simulink model "receiver_overall_reset"  (Simulink 7.5)
settings: Solver=FixedStepDiscrete  SolverMode=SingleTasking  StartTime=0.0  StopTime=(length(simin.signals.values)-1)/Fs  FixedStep=1  RelTol=1e-3
undefined symbols (not defined in the file): Fs
libraries: xbsIndex_r4 x962
(part 9 of 9)

== system receiver_overall_reset/Receiver/Sym-Chooser/3-11/Corr0/Delay_Line/DE14/1to2 ==
  In : Inport  OutDataType=fixdt(1, 16)  OutScaling=2^0
  Out1 : Outport  OutDataType=fixdt(1, 16)  OutScaling=2^0
  Out2 : Outport  Port=2  OutDataType=fixdt(1, 16)  OutScaling=2^0
  wires:
  In/1 -> Out2/1, Out1/1

== system receiver_overall_reset/Receiver/Sym-Chooser/3-11/Corr0/Delay_Line/DE15/1to2 ==
  In : Inport  OutDataType=fixdt(1, 16)  OutScaling=2^0
  Out1 : Outport  OutDataType=fixdt(1, 16)  OutScaling=2^0
  Out2 : Outport  Port=2  OutDataType=fixdt(1, 16)  OutScaling=2^0
  wires:
  In/1 -> Out2/1, Out1/1

== system receiver_overall_reset/Receiver/Sym-Chooser/3-11/Corr0/Delay_Line/DE16/1to2 ==
  In : Inport  OutDataType=fixdt(1, 16)  OutScaling=2^0
  Out1 : Outport  OutDataType=fixdt(1, 16)  OutScaling=2^0
  Out2 : Outport  Port=2  OutDataType=fixdt(1, 16)  OutScaling=2^0
  wires:
  In/1 -> Out2/1, Out1/1

== system receiver_overall_reset/Receiver/Sym-Chooser/3-11/Corr0/Delay_Line/DE17/1to2 ==
  In : Inport  OutDataType=fixdt(1, 16)  OutScaling=2^0
  Out1 : Outport  OutDataType=fixdt(1, 16)  OutScaling=2^0
  Out2 : Outport  Port=2  OutDataType=fixdt(1, 16)  OutScaling=2^0
  wires:
  In/1 -> Out2/1, Out1/1

== system receiver_overall_reset/Receiver/Sym-Chooser/3-11/Corr0/Delay_Line/DE18/1to2 ==
  In : Inport  OutDataType=fixdt(1, 16)  OutScaling=2^0
  Out1 : Outport  OutDataType=fixdt(1, 16)  OutScaling=2^0
  Out2 : Outport  Port=2  OutDataType=fixdt(1, 16)  OutScaling=2^0
  wires:
  In/1 -> Out2/1, Out1/1

== system receiver_overall_reset/Receiver/Sym-Chooser/3-11/Corr0/Delay_Line/DE19/1to2 ==
  In : Inport  OutDataType=fixdt(1, 16)  OutScaling=2^0
  Out1 : Outport  OutDataType=fixdt(1, 16)  OutScaling=2^0
  Out2 : Outport  Port=2  OutDataType=fixdt(1, 16)  OutScaling=2^0
  wires:
  In/1 -> Out2/1, Out1/1

== system receiver_overall_reset/Receiver/Sym-Chooser/3-11/Corr0/Delay_Line/DE2/1to2 ==
  In : Inport  OutDataType=fixdt(1, 16)  OutScaling=2^0
  Out1 : Outport  OutDataType=fixdt(1, 16)  OutScaling=2^0
  Out2 : Outport  Port=2  OutDataType=fixdt(1, 16)  OutScaling=2^0
  wires:
  In/1 -> Out2/1, Out1/1

== system receiver_overall_reset/Receiver/Sym-Chooser/3-11/Corr0/Delay_Line/DE20/1to2 ==
  In : Inport  OutDataType=fixdt(1, 16)  OutScaling=2^0
  Out1 : Outport  OutDataType=fixdt(1, 16)  OutScaling=2^0
  Out2 : Outport  Port=2  OutDataType=fixdt(1, 16)  OutScaling=2^0
  wires:
  In/1 -> Out2/1, Out1/1

== system receiver_overall_reset/Receiver/Sym-Chooser/3-11/Corr0/Delay_Line/DE21/1to2 ==
  In : Inport  OutDataType=fixdt(1, 16)  OutScaling=2^0
  Out1 : Outport  OutDataType=fixdt(1, 16)  OutScaling=2^0
  Out2 : Outport  Port=2  OutDataType=fixdt(1, 16)  OutScaling=2^0
  wires:
  In/1 -> Out2/1, Out1/1

== system receiver_overall_reset/Receiver/Sym-Chooser/3-11/Corr0/Delay_Line/DE22/1to2 ==
  In : Inport  OutDataType=fixdt(1, 16)  OutScaling=2^0
  Out1 : Outport  OutDataType=fixdt(1, 16)  OutScaling=2^0
  Out2 : Outport  Port=2  OutDataType=fixdt(1, 16)  OutScaling=2^0
  wires:
  In/1 -> Out2/1, Out1/1

== system receiver_overall_reset/Receiver/Sym-Chooser/3-11/Corr0/Delay_Line/DE23/1to2 ==
  In : Inport  OutDataType=fixdt(1, 16)  OutScaling=2^0
  Out1 : Outport  OutDataType=fixdt(1, 16)  OutScaling=2^0
  Out2 : Outport  Port=2  OutDataType=fixdt(1, 16)  OutScaling=2^0
  wires:
  In/1 -> Out2/1, Out1/1

== system receiver_overall_reset/Receiver/Sym-Chooser/3-11/Corr0/Delay_Line/DE24/1to2 ==
  In : Inport  OutDataType=fixdt(1, 16)  OutScaling=2^0
  Out1 : Outport  OutDataType=fixdt(1, 16)  OutScaling=2^0
  Out2 : Outport  Port=2  OutDataType=fixdt(1, 16)  OutScaling=2^0
  wires:
  In/1 -> Out2/1, Out1/1

== system receiver_overall_reset/Receiver/Sym-Chooser/3-11/Corr0/Delay_Line/DE25/1to2 ==
  In : Inport  OutDataType=fixdt(1, 16)  OutScaling=2^0
  Out1 : Outport  OutDataType=fixdt(1, 16)  OutScaling=2^0
  Out2 : Outport  Port=2  OutDataType=fixdt(1, 16)  OutScaling=2^0
  wires:
  In/1 -> Out2/1, Out1/1

== system receiver_overall_reset/Receiver/Sym-Chooser/3-11/Corr0/Delay_Line/DE26/1to2 ==
  In : Inport  OutDataType=fixdt(1, 16)  OutScaling=2^0
  Out1 : Outport  OutDataType=fixdt(1, 16)  OutScaling=2^0
  Out2 : Outport  Port=2  OutDataType=fixdt(1, 16)  OutScaling=2^0
  wires:
  In/1 -> Out2/1, Out1/1

== system receiver_overall_reset/Receiver/Sym-Chooser/3-11/Corr0/Delay_Line/DE27/1to2 ==
  In : Inport  OutDataType=fixdt(1, 16)  OutScaling=2^0
  Out1 : Outport  OutDataType=fixdt(1, 16)  OutScaling=2^0
  Out2 : Outport  Port=2  OutDataType=fixdt(1, 16)  OutScaling=2^0
  wires:
  In/1 -> Out2/1, Out1/1

== system receiver_overall_reset/Receiver/Sym-Chooser/3-11/Corr0/Delay_Line/DE28/1to2 ==
  In : Inport  OutDataType=fixdt(1, 16)  OutScaling=2^0
  Out1 : Outport  OutDataType=fixdt(1, 16)  OutScaling=2^0
  Out2 : Outport  Port=2  OutDataType=fixdt(1, 16)  OutScaling=2^0
  wires:
  In/1 -> Out2/1, Out1/1

== system receiver_overall_reset/Receiver/Sym-Chooser/3-11/Corr0/Delay_Line/DE29/1to2 ==
  In : Inport  OutDataType=fixdt(1, 16)  OutScaling=2^0
  Out1 : Outport  OutDataType=fixdt(1, 16)  OutScaling=2^0
  Out2 : Outport  Port=2  OutDataType=fixdt(1, 16)  OutScaling=2^0
  wires:
  In/1 -> Out2/1, Out1/1

== system receiver_overall_reset/Receiver/Sym-Chooser/3-11/Corr0/Delay_Line/DE3/1to2 ==
  In : Inport  OutDataType=fixdt(1, 16)  OutScaling=2^0
  Out1 : Outport  OutDataType=fixdt(1, 16)  OutScaling=2^0
  Out2 : Outport  Port=2  OutDataType=fixdt(1, 16)  OutScaling=2^0
  wires:
  In/1 -> Out2/1, Out1/1

== system receiver_overall_reset/Receiver/Sym-Chooser/3-11/Corr0/Delay_Line/DE30/1to2 ==
  In : Inport  OutDataType=fixdt(1, 16)  OutScaling=2^0
  Out1 : Outport  OutDataType=fixdt(1, 16)  OutScaling=2^0
  Out2 : Outport  Port=2  OutDataType=fixdt(1, 16)  OutScaling=2^0
  wires:
  In/1 -> Out2/1, Out1/1

== system receiver_overall_reset/Receiver/Sym-Chooser/3-11/Corr0/Delay_Line/DE4/1to2 ==
  In : Inport  OutDataType=fixdt(1, 16)  OutScaling=2^0
  Out1 : Outport  OutDataType=fixdt(1, 16)  OutScaling=2^0
  Out2 : Outport  Port=2  OutDataType=fixdt(1, 16)  OutScaling=2^0
  wires:
  In/1 -> Out2/1, Out1/1

== system receiver_overall_reset/Receiver/Sym-Chooser/3-11/Corr0/Delay_Line/DE5/1to2 ==
  In : Inport  OutDataType=fixdt(1, 16)  OutScaling=2^0
  Out1 : Outport  OutDataType=fixdt(1, 16)  OutScaling=2^0
  Out2 : Outport  Port=2  OutDataType=fixdt(1, 16)  OutScaling=2^0
  wires:
  In/1 -> Out2/1, Out1/1

== system receiver_overall_reset/Receiver/Sym-Chooser/3-11/Corr0/Delay_Line/DE6/1to2 ==
  In : Inport  OutDataType=fixdt(1, 16)  OutScaling=2^0
  Out1 : Outport  OutDataType=fixdt(1, 16)  OutScaling=2^0
  Out2 : Outport  Port=2  OutDataType=fixdt(1, 16)  OutScaling=2^0
  wires:
  In/1 -> Out2/1, Out1/1

== system receiver_overall_reset/Receiver/Sym-Chooser/3-11/Corr0/Delay_Line/DE7/1to2 ==
  In : Inport  OutDataType=fixdt(1, 16)  OutScaling=2^0
  Out1 : Outport  OutDataType=fixdt(1, 16)  OutScaling=2^0
  Out2 : Outport  Port=2  OutDataType=fixdt(1, 16)  OutScaling=2^0
  wires:
  In/1 -> Out2/1, Out1/1

== system receiver_overall_reset/Receiver/Sym-Chooser/3-11/Corr0/Delay_Line/DE8/1to2 ==
  In : Inport  OutDataType=fixdt(1, 16)  OutScaling=2^0
  Out1 : Outport  OutDataType=fixdt(1, 16)  OutScaling=2^0
  Out2 : Outport  Port=2  OutDataType=fixdt(1, 16)  OutScaling=2^0
  wires:
  In/1 -> Out2/1, Out1/1

== system receiver_overall_reset/Receiver/Sym-Chooser/3-11/Corr0/Delay_Line/DE9/1to2 ==
  In : Inport  OutDataType=fixdt(1, 16)  OutScaling=2^0
  Out1 : Outport  OutDataType=fixdt(1, 16)  OutScaling=2^0
  Out2 : Outport  Port=2  OutDataType=fixdt(1, 16)  OutScaling=2^0
  wires:
  In/1 -> Out2/1, Out1/1

== system receiver_overall_reset/Receiver/Sym-Chooser/4-12/Corr0/Delay_Line/DE1/1to2 ==
  In : Inport  OutDataType=fixdt(1, 16)  OutScaling=2^0
  Out1 : Outport  OutDataType=fixdt(1, 16)  OutScaling=2^0
  Out2 : Outport  Port=2  OutDataType=fixdt(1, 16)  OutScaling=2^0
  wires:
  In/1 -> Out1/1, Out2/1

== system receiver_overall_reset/Receiver/Sym-Chooser/4-12/Corr0/Delay_Line/DE10/1to2 ==
  In : Inport  OutDataType=fixdt(1, 16)  OutScaling=2^0
  Out1 : Outport  OutDataType=fixdt(1, 16)  OutScaling=2^0
  Out2 : Outport  Port=2  OutDataType=fixdt(1, 16)  OutScaling=2^0
  wires:
  In/1 -> Out2/1, Out1/1

== system receiver_overall_reset/Receiver/Sym-Chooser/4-12/Corr0/Delay_Line/DE11/1to2 ==
  In : Inport  OutDataType=fixdt(1, 16)  OutScaling=2^0
  Out1 : Outport  OutDataType=fixdt(1, 16)  OutScaling=2^0
  Out2 : Outport  Port=2  OutDataType=fixdt(1, 16)  OutScaling=2^0
  wires:
  In/1 -> Out2/1, Out1/1

== system receiver_overall_reset/Receiver/Sym-Chooser/4-12/Corr0/Delay_Line/DE12/1to2 ==
  In : Inport  OutDataType=fixdt(1, 16)  OutScaling=2^0
  Out1 : Outport  OutDataType=fixdt(1, 16)  OutScaling=2^0
  Out2 : Outport  Port=2  OutDataType=fixdt(1, 16)  OutScaling=2^0
  wires:
  In/1 -> Out2/1, Out1/1

== system receiver_overall_reset/Receiver/Sym-Chooser/4-12/Corr0/Delay_Line/DE13/1to2 ==
  In : Inport  OutDataType=fixdt(1, 16)  OutScaling=2^0
  Out1 : Outport  OutDataType=fixdt(1, 16)  OutScaling=2^0
  Out2 : Outport  Port=2  OutDataType=fixdt(1, 16)  OutScaling=2^0
  wires:
  In/1 -> Out2/1, Out1/1

== system receiver_overall_reset/Receiver/Sym-Chooser/4-12/Corr0/Delay_Line/DE14/1to2 ==
  In : Inport  OutDataType=fixdt(1, 16)  OutScaling=2^0
  Out1 : Outport  OutDataType=fixdt(1, 16)  OutScaling=2^0
  Out2 : Outport  Port=2  OutDataType=fixdt(1, 16)  OutScaling=2^0
  wires:
  In/1 -> Out2/1, Out1/1

== system receiver_overall_reset/Receiver/Sym-Chooser/4-12/Corr0/Delay_Line/DE15/1to2 ==
  In : Inport  OutDataType=fixdt(1, 16)  OutScaling=2^0
  Out1 : Outport  OutDataType=fixdt(1, 16)  OutScaling=2^0
  Out2 : Outport  Port=2  OutDataType=fixdt(1, 16)  OutScaling=2^0
  wires:
  In/1 -> Out2/1, Out1/1

== system receiver_overall_reset/Receiver/Sym-Chooser/4-12/Corr0/Delay_Line/DE16/1to2 ==
  In : Inport  OutDataType=fixdt(1, 16)  OutScaling=2^0
  Out1 : Outport  OutDataType=fixdt(1, 16)  OutScaling=2^0
  Out2 : Outport  Port=2  OutDataType=fixdt(1, 16)  OutScaling=2^0
  wires:
  In/1 -> Out2/1, Out1/1

== system receiver_overall_reset/Receiver/Sym-Chooser/4-12/Corr0/Delay_Line/DE17/1to2 ==
  In : Inport  OutDataType=fixdt(1, 16)  OutScaling=2^0
  Out1 : Outport  OutDataType=fixdt(1, 16)  OutScaling=2^0
  Out2 : Outport  Port=2  OutDataType=fixdt(1, 16)  OutScaling=2^0
  wires:
  In/1 -> Out2/1, Out1/1

== system receiver_overall_reset/Receiver/Sym-Chooser/4-12/Corr0/Delay_Line/DE18/1to2 ==
  In : Inport  OutDataType=fixdt(1, 16)  OutScaling=2^0
  Out1 : Outport  OutDataType=fixdt(1, 16)  OutScaling=2^0
  Out2 : Outport  Port=2  OutDataType=fixdt(1, 16)  OutScaling=2^0
  wires:
  In/1 -> Out2/1, Out1/1

== system receiver_overall_reset/Receiver/Sym-Chooser/4-12/Corr0/Delay_Line/DE19/1to2 ==
  In : Inport  OutDataType=fixdt(1, 16)  OutScaling=2^0
  Out1 : Outport  OutDataType=fixdt(1, 16)  OutScaling=2^0
  Out2 : Outport  Port=2  OutDataType=fixdt(1, 16)  OutScaling=2^0
  wires:
  In/1 -> Out2/1, Out1/1

== system receiver_overall_reset/Receiver/Sym-Chooser/4-12/Corr0/Delay_Line/DE2/1to2 ==
  In : Inport  OutDataType=fixdt(1, 16)  OutScaling=2^0
  Out1 : Outport  OutDataType=fixdt(1, 16)  OutScaling=2^0
  Out2 : Outport  Port=2  OutDataType=fixdt(1, 16)  OutScaling=2^0
  wires:
  In/1 -> Out2/1, Out1/1

== system receiver_overall_reset/Receiver/Sym-Chooser/4-12/Corr0/Delay_Line/DE20/1to2 ==
  In : Inport  OutDataType=fixdt(1, 16)  OutScaling=2^0
  Out1 : Outport  OutDataType=fixdt(1, 16)  OutScaling=2^0
  Out2 : Outport  Port=2  OutDataType=fixdt(1, 16)  OutScaling=2^0
  wires:
  In/1 -> Out2/1, Out1/1

== system receiver_overall_reset/Receiver/Sym-Chooser/4-12/Corr0/Delay_Line/DE21/1to2 ==
  In : Inport  OutDataType=fixdt(1, 16)  OutScaling=2^0
  Out1 : Outport  OutDataType=fixdt(1, 16)  OutScaling=2^0
  Out2 : Outport  Port=2  OutDataType=fixdt(1, 16)  OutScaling=2^0
  wires:
  In/1 -> Out2/1, Out1/1

== system receiver_overall_reset/Receiver/Sym-Chooser/4-12/Corr0/Delay_Line/DE22/1to2 ==
  In : Inport  OutDataType=fixdt(1, 16)  OutScaling=2^0
  Out1 : Outport  OutDataType=fixdt(1, 16)  OutScaling=2^0
  Out2 : Outport  Port=2  OutDataType=fixdt(1, 16)  OutScaling=2^0
  wires:
  In/1 -> Out2/1, Out1/1

== system receiver_overall_reset/Receiver/Sym-Chooser/4-12/Corr0/Delay_Line/DE23/1to2 ==
  In : Inport  OutDataType=fixdt(1, 16)  OutScaling=2^0
  Out1 : Outport  OutDataType=fixdt(1, 16)  OutScaling=2^0
  Out2 : Outport  Port=2  OutDataType=fixdt(1, 16)  OutScaling=2^0
  wires:
  In/1 -> Out2/1, Out1/1

== system receiver_overall_reset/Receiver/Sym-Chooser/4-12/Corr0/Delay_Line/DE24/1to2 ==
  In : Inport  OutDataType=fixdt(1, 16)  OutScaling=2^0
  Out1 : Outport  OutDataType=fixdt(1, 16)  OutScaling=2^0
  Out2 : Outport  Port=2  OutDataType=fixdt(1, 16)  OutScaling=2^0
  wires:
  In/1 -> Out2/1, Out1/1

== system receiver_overall_reset/Receiver/Sym-Chooser/4-12/Corr0/Delay_Line/DE25/1to2 ==
  In : Inport  OutDataType=fixdt(1, 16)  OutScaling=2^0
  Out1 : Outport  OutDataType=fixdt(1, 16)  OutScaling=2^0
  Out2 : Outport  Port=2  OutDataType=fixdt(1, 16)  OutScaling=2^0
  wires:
  In/1 -> Out2/1, Out1/1

== system receiver_overall_reset/Receiver/Sym-Chooser/4-12/Corr0/Delay_Line/DE26/1to2 ==
  In : Inport  OutDataType=fixdt(1, 16)  OutScaling=2^0
  Out1 : Outport  OutDataType=fixdt(1, 16)  OutScaling=2^0
  Out2 : Outport  Port=2  OutDataType=fixdt(1, 16)  OutScaling=2^0
  wires:
  In/1 -> Out2/1, Out1/1

== system receiver_overall_reset/Receiver/Sym-Chooser/4-12/Corr0/Delay_Line/DE27/1to2 ==
  In : Inport  OutDataType=fixdt(1, 16)  OutScaling=2^0
  Out1 : Outport  OutDataType=fixdt(1, 16)  OutScaling=2^0
  Out2 : Outport  Port=2  OutDataType=fixdt(1, 16)  OutScaling=2^0
  wires:
  In/1 -> Out2/1, Out1/1

== system receiver_overall_reset/Receiver/Sym-Chooser/4-12/Corr0/Delay_Line/DE28/1to2 ==
  In : Inport  OutDataType=fixdt(1, 16)  OutScaling=2^0
  Out1 : Outport  OutDataType=fixdt(1, 16)  OutScaling=2^0
  Out2 : Outport  Port=2  OutDataType=fixdt(1, 16)  OutScaling=2^0
  wires:
  In/1 -> Out2/1, Out1/1

== system receiver_overall_reset/Receiver/Sym-Chooser/4-12/Corr0/Delay_Line/DE29/1to2 ==
  In : Inport  OutDataType=fixdt(1, 16)  OutScaling=2^0
  Out1 : Outport  OutDataType=fixdt(1, 16)  OutScaling=2^0
  Out2 : Outport  Port=2  OutDataType=fixdt(1, 16)  OutScaling=2^0
  wires:
  In/1 -> Out2/1, Out1/1

== system receiver_overall_reset/Receiver/Sym-Chooser/4-12/Corr0/Delay_Line/DE3/1to2 ==
  In : Inport  OutDataType=fixdt(1, 16)  OutScaling=2^0
  Out1 : Outport  OutDataType=fixdt(1, 16)  OutScaling=2^0
  Out2 : Outport  Port=2  OutDataType=fixdt(1, 16)  OutScaling=2^0
  wires:
  In/1 -> Out2/1, Out1/1

== system receiver_overall_reset/Receiver/Sym-Chooser/4-12/Corr0/Delay_Line/DE30/1to2 ==
  In : Inport  OutDataType=fixdt(1, 16)  OutScaling=2^0
  Out1 : Outport  OutDataType=fixdt(1, 16)  OutScaling=2^0
  Out2 : Outport  Port=2  OutDataType=fixdt(1, 16)  OutScaling=2^0
  wires:
  In/1 -> Out2/1, Out1/1

== system receiver_overall_reset/Receiver/Sym-Chooser/4-12/Corr0/Delay_Line/DE4/1to2 ==
  In : Inport  OutDataType=fixdt(1, 16)  OutScaling=2^0
  Out1 : Outport  OutDataType=fixdt(1, 16)  OutScaling=2^0
  Out2 : Outport  Port=2  OutDataType=fixdt(1, 16)  OutScaling=2^0
  wires:
  In/1 -> Out2/1, Out1/1

== system receiver_overall_reset/Receiver/Sym-Chooser/4-12/Corr0/Delay_Line/DE5/1to2 ==
  In : Inport  OutDataType=fixdt(1, 16)  OutScaling=2^0
  Out1 : Outport  OutDataType=fixdt(1, 16)  OutScaling=2^0
  Out2 : Outport  Port=2  OutDataType=fixdt(1, 16)  OutScaling=2^0
  wires:
  In/1 -> Out2/1, Out1/1

== system receiver_overall_reset/Receiver/Sym-Chooser/4-12/Corr0/Delay_Line/DE6/1to2 ==
  In : Inport  OutDataType=fixdt(1, 16)  OutScaling=2^0
  Out1 : Outport  OutDataType=fixdt(1, 16)  OutScaling=2^0
  Out2 : Outport  Port=2  OutDataType=fixdt(1, 16)  OutScaling=2^0
  wires:
  In/1 -> Out2/1, Out1/1

== system receiver_overall_reset/Receiver/Sym-Chooser/4-12/Corr0/Delay_Line/DE7/1to2 ==
  In : Inport  OutDataType=fixdt(1, 16)  OutScaling=2^0
  Out1 : Outport  OutDataType=fixdt(1, 16)  OutScaling=2^0
  Out2 : Outport  Port=2  OutDataType=fixdt(1, 16)  OutScaling=2^0
  wires:
  In/1 -> Out2/1, Out1/1

== system receiver_overall_reset/Receiver/Sym-Chooser/4-12/Corr0/Delay_Line/DE8/1to2 ==
  In : Inport  OutDataType=fixdt(1, 16)  OutScaling=2^0
  Out1 : Outport  OutDataType=fixdt(1, 16)  OutScaling=2^0
  Out2 : Outport  Port=2  OutDataType=fixdt(1, 16)  OutScaling=2^0
  wires:
  In/1 -> Out2/1, Out1/1

== system receiver_overall_reset/Receiver/Sym-Chooser/4-12/Corr0/Delay_Line/DE9/1to2 ==
  In : Inport  OutDataType=fixdt(1, 16)  OutScaling=2^0
  Out1 : Outport  OutDataType=fixdt(1, 16)  OutScaling=2^0
  Out2 : Outport  Port=2  OutDataType=fixdt(1, 16)  OutScaling=2^0
  wires:
  In/1 -> Out2/1, Out1/1

== system receiver_overall_reset/Receiver/Sym-Chooser/5-13/Corr0/Delay_Line/DE1/1to2 ==
  In : Inport  OutDataType=fixdt(1, 16)  OutScaling=2^0
  Out1 : Outport  OutDataType=fixdt(1, 16)  OutScaling=2^0
  Out2 : Outport  Port=2  OutDataType=fixdt(1, 16)  OutScaling=2^0
  wires:
  In/1 -> Out1/1, Out2/1

== system receiver_overall_reset/Receiver/Sym-Chooser/5-13/Corr0/Delay_Line/DE10/1to2 ==
  In : Inport  OutDataType=fixdt(1, 16)  OutScaling=2^0
  Out1 : Outport  OutDataType=fixdt(1, 16)  OutScaling=2^0
  Out2 : Outport  Port=2  OutDataType=fixdt(1, 16)  OutScaling=2^0
  wires:
  In/1 -> Out2/1, Out1/1

== system receiver_overall_reset/Receiver/Sym-Chooser/5-13/Corr0/Delay_Line/DE11/1to2 ==
  In : Inport  OutDataType=fixdt(1, 16)  OutScaling=2^0
  Out1 : Outport  OutDataType=fixdt(1, 16)  OutScaling=2^0
  Out2 : Outport  Port=2  OutDataType=fixdt(1, 16)  OutScaling=2^0
  wires:
  In/1 -> Out2/1, Out1/1

== system receiver_overall_reset/Receiver/Sym-Chooser/5-13/Corr0/Delay_Line/DE12/1to2 ==
  In : Inport  OutDataType=fixdt(1, 16)  OutScaling=2^0
  Out1 : Outport  OutDataType=fixdt(1, 16)  OutScaling=2^0
  Out2 : Outport  Port=2  OutDataType=fixdt(1, 16)  OutScaling=2^0
  wires:
  In/1 -> Out2/1, Out1/1

== system receiver_overall_reset/Receiver/Sym-Chooser/5-13/Corr0/Delay_Line/DE13/1to2 ==
  In : Inport  OutDataType=fixdt(1, 16)  OutScaling=2^0
  Out1 : Outport  OutDataType=fixdt(1, 16)  OutScaling=2^0
  Out2 : Outport  Port=2  OutDataType=fixdt(1, 16)  OutScaling=2^0
  wires:
  In/1 -> Out2/1, Out1/1

== system receiver_overall_reset/Receiver/Sym-Chooser/5-13/Corr0/Delay_Line/DE14/1to2 ==
  In : Inport  OutDataType=fixdt(1, 16)  OutScaling=2^0
  Out1 : Outport  OutDataType=fixdt(1, 16)  OutScaling=2^0
  Out2 : Outport  Port=2  OutDataType=fixdt(1, 16)  OutScaling=2^0
  wires:
  In/1 -> Out2/1, Out1/1

== system receiver_overall_reset/Receiver/Sym-Chooser/5-13/Corr0/Delay_Line/DE15/1to2 ==
  In : Inport  OutDataType=fixdt(1, 16)  OutScaling=2^0
  Out1 : Outport  OutDataType=fixdt(1, 16)  OutScaling=2^0
  Out2 : Outport  Port=2  OutDataType=fixdt(1, 16)  OutScaling=2^0
  wires:
  In/1 -> Out2/1, Out1/1

== system receiver_overall_reset/Receiver/Sym-Chooser/5-13/Corr0/Delay_Line/DE16/1to2 ==
  In : Inport  OutDataType=fixdt(1, 16)  OutScaling=2^0
  Out1 : Outport  OutDataType=fixdt(1, 16)  OutScaling=2^0
  Out2 : Outport  Port=2  OutDataType=fixdt(1, 16)  OutScaling=2^0
  wires:
  In/1 -> Out2/1, Out1/1

== system receiver_overall_reset/Receiver/Sym-Chooser/5-13/Corr0/Delay_Line/DE17/1to2 ==
  In : Inport  OutDataType=fixdt(1, 16)  OutScaling=2^0
  Out1 : Outport  OutDataType=fixdt(1, 16)  OutScaling=2^0
  Out2 : Outport  Port=2  OutDataType=fixdt(1, 16)  OutScaling=2^0
  wires:
  In/1 -> Out2/1, Out1/1

== system receiver_overall_reset/Receiver/Sym-Chooser/5-13/Corr0/Delay_Line/DE18/1to2 ==
  In : Inport  OutDataType=fixdt(1, 16)  OutScaling=2^0
  Out1 : Outport  OutDataType=fixdt(1, 16)  OutScaling=2^0
  Out2 : Outport  Port=2  OutDataType=fixdt(1, 16)  OutScaling=2^0
  wires:
  In/1 -> Out2/1, Out1/1

== system receiver_overall_reset/Receiver/Sym-Chooser/5-13/Corr0/Delay_Line/DE19/1to2 ==
  In : Inport  OutDataType=fixdt(1, 16)  OutScaling=2^0
  Out1 : Outport  OutDataType=fixdt(1, 16)  OutScaling=2^0
  Out2 : Outport  Port=2  OutDataType=fixdt(1, 16)  OutScaling=2^0
  wires:
  In/1 -> Out2/1, Out1/1

== system receiver_overall_reset/Receiver/Sym-Chooser/5-13/Corr0/Delay_Line/DE2/1to2 ==
  In : Inport  OutDataType=fixdt(1, 16)  OutScaling=2^0
  Out1 : Outport  OutDataType=fixdt(1, 16)  OutScaling=2^0
  Out2 : Outport  Port=2  OutDataType=fixdt(1, 16)  OutScaling=2^0
  wires:
  In/1 -> Out2/1, Out1/1

== system receiver_overall_reset/Receiver/Sym-Chooser/5-13/Corr0/Delay_Line/DE20/1to2 ==
  In : Inport  OutDataType=fixdt(1, 16)  OutScaling=2^0
  Out1 : Outport  OutDataType=fixdt(1, 16)  OutScaling=2^0
  Out2 : Outport  Port=2  OutDataType=fixdt(1, 16)  OutScaling=2^0
  wires:
  In/1 -> Out2/1, Out1/1

== system receiver_overall_reset/Receiver/Sym-Chooser/5-13/Corr0/Delay_Line/DE21/1to2 ==
  In : Inport  OutDataType=fixdt(1, 16)  OutScaling=2^0
  Out1 : Outport  OutDataType=fixdt(1, 16)  OutScaling=2^0
  Out2 : Outport  Port=2  OutDataType=fixdt(1, 16)  OutScaling=2^0
  wires:
  In/1 -> Out2/1, Out1/1

== system receiver_overall_reset/Receiver/Sym-Chooser/5-13/Corr0/Delay_Line/DE22/1to2 ==
  In : Inport  OutDataType=fixdt(1, 16)  OutScaling=2^0
  Out1 : Outport  OutDataType=fixdt(1, 16)  OutScaling=2^0
  Out2 : Outport  Port=2  OutDataType=fixdt(1, 16)  OutScaling=2^0
  wires:
  In/1 -> Out2/1, Out1/1

== system receiver_overall_reset/Receiver/Sym-Chooser/5-13/Corr0/Delay_Line/DE23/1to2 ==
  In : Inport  OutDataType=fixdt(1, 16)  OutScaling=2^0
  Out1 : Outport  OutDataType=fixdt(1, 16)  OutScaling=2^0
  Out2 : Outport  Port=2  OutDataType=fixdt(1, 16)  OutScaling=2^0
  wires:
  In/1 -> Out2/1, Out1/1

== system receiver_overall_reset/Receiver/Sym-Chooser/5-13/Corr0/Delay_Line/DE24/1to2 ==
  In : Inport  OutDataType=fixdt(1, 16)  OutScaling=2^0
  Out1 : Outport  OutDataType=fixdt(1, 16)  OutScaling=2^0
  Out2 : Outport  Port=2  OutDataType=fixdt(1, 16)  OutScaling=2^0
  wires:
  In/1 -> Out2/1, Out1/1

== system receiver_overall_reset/Receiver/Sym-Chooser/5-13/Corr0/Delay_Line/DE25/1to2 ==
  In : Inport  OutDataType=fixdt(1, 16)  OutScaling=2^0
  Out1 : Outport  OutDataType=fixdt(1, 16)  OutScaling=2^0
  Out2 : Outport  Port=2  OutDataType=fixdt(1, 16)  OutScaling=2^0
  wires:
  In/1 -> Out2/1, Out1/1

== system receiver_overall_reset/Receiver/Sym-Chooser/5-13/Corr0/Delay_Line/DE26/1to2 ==
  In : Inport  OutDataType=fixdt(1, 16)  OutScaling=2^0
  Out1 : Outport  OutDataType=fixdt(1, 16)  OutScaling=2^0
  Out2 : Outport  Port=2  OutDataType=fixdt(1, 16)  OutScaling=2^0
  wires:
  In/1 -> Out2/1, Out1/1

== system receiver_overall_reset/Receiver/Sym-Chooser/5-13/Corr0/Delay_Line/DE27/1to2 ==
  In : Inport  OutDataType=fixdt(1, 16)  OutScaling=2^0
  Out1 : Outport  OutDataType=fixdt(1, 16)  OutScaling=2^0
  Out2 : Outport  Port=2  OutDataType=fixdt(1, 16)  OutScaling=2^0
  wires:
  In/1 -> Out2/1, Out1/1

== system receiver_overall_reset/Receiver/Sym-Chooser/5-13/Corr0/Delay_Line/DE28/1to2 ==
  In : Inport  OutDataType=fixdt(1, 16)  OutScaling=2^0
  Out1 : Outport  OutDataType=fixdt(1, 16)  OutScaling=2^0
  Out2 : Outport  Port=2  OutDataType=fixdt(1, 16)  OutScaling=2^0
  wires:
  In/1 -> Out2/1, Out1/1

== system receiver_overall_reset/Receiver/Sym-Chooser/5-13/Corr0/Delay_Line/DE29/1to2 ==
  In : Inport  OutDataType=fixdt(1, 16)  OutScaling=2^0
  Out1 : Outport  OutDataType=fixdt(1, 16)  OutScaling=2^0
  Out2 : Outport  Port=2  OutDataType=fixdt(1, 16)  OutScaling=2^0
  wires:
  In/1 -> Out2/1, Out1/1

== system receiver_overall_reset/Receiver/Sym-Chooser/5-13/Corr0/Delay_Line/DE3/1to2 ==
  In : Inport  OutDataType=fixdt(1, 16)  OutScaling=2^0
  Out1 : Outport  OutDataType=fixdt(1, 16)  OutScaling=2^0
  Out2 : Outport  Port=2  OutDataType=fixdt(1, 16)  OutScaling=2^0
  wires:
  In/1 -> Out2/1, Out1/1

== system receiver_overall_reset/Receiver/Sym-Chooser/5-13/Corr0/Delay_Line/DE30/1to2 ==
  In : Inport  OutDataType=fixdt(1, 16)  OutScaling=2^0
  Out1 : Outport  OutDataType=fixdt(1, 16)  OutScaling=2^0
  Out2 : Outport  Port=2  OutDataType=fixdt(1, 16)  OutScaling=2^0
  wires:
  In/1 -> Out2/1, Out1/1

== system receiver_overall_reset/Receiver/Sym-Chooser/5-13/Corr0/Delay_Line/DE4/1to2 ==
  In : Inport  OutDataType=fixdt(1, 16)  OutScaling=2^0
  Out1 : Outport  OutDataType=fixdt(1, 16)  OutScaling=2^0
  Out2 : Outport  Port=2  OutDataType=fixdt(1, 16)  OutScaling=2^0
  wires:
  In/1 -> Out2/1, Out1/1

== system receiver_overall_reset/Receiver/Sym-Chooser/5-13/Corr0/Delay_Line/DE5/1to2 ==
  In : Inport  OutDataType=fixdt(1, 16)  OutScaling=2^0
  Out1 : Outport  OutDataType=fixdt(1, 16)  OutScaling=2^0
  Out2 : Outport  Port=2  OutDataType=fixdt(1, 16)  OutScaling=2^0
  wires:
  In/1 -> Out2/1, Out1/1

== system receiver_overall_reset/Receiver/Sym-Chooser/5-13/Corr0/Delay_Line/DE6/1to2 ==
  In : Inport  OutDataType=fixdt(1, 16)  OutScaling=2^0
  Out1 : Outport  OutDataType=fixdt(1, 16)  OutScaling=2^0
  Out2 : Outport  Port=2  OutDataType=fixdt(1, 16)  OutScaling=2^0
  wires:
  In/1 -> Out2/1, Out1/1

== system receiver_overall_reset/Receiver/Sym-Chooser/5-13/Corr0/Delay_Line/DE7/1to2 ==
  In : Inport  OutDataType=fixdt(1, 16)  OutScaling=2^0
  Out1 : Outport  OutDataType=fixdt(1, 16)  OutScaling=2^0
  Out2 : Outport  Port=2  OutDataType=fixdt(1, 16)  OutScaling=2^0
  wires:
  In/1 -> Out2/1, Out1/1

== system receiver_overall_reset/Receiver/Sym-Chooser/5-13/Corr0/Delay_Line/DE8/1to2 ==
  In : Inport  OutDataType=fixdt(1, 16)  OutScaling=2^0
  Out1 : Outport  OutDataType=fixdt(1, 16)  OutScaling=2^0
  Out2 : Outport  Port=2  OutDataType=fixdt(1, 16)  OutScaling=2^0
  wires:
  In/1 -> Out2/1, Out1/1

== system receiver_overall_reset/Receiver/Sym-Chooser/5-13/Corr0/Delay_Line/DE9/1to2 ==
  In : Inport  OutDataType=fixdt(1, 16)  OutScaling=2^0
  Out1 : Outport  OutDataType=fixdt(1, 16)  OutScaling=2^0
  Out2 : Outport  Port=2  OutDataType=fixdt(1, 16)  OutScaling=2^0
  wires:
  In/1 -> Out2/1, Out1/1

== system receiver_overall_reset/Receiver/Sym-Chooser/6-14/Corr0/Delay_Line/DE1/1to2 ==
  In : Inport  OutDataType=fixdt(1, 16)  OutScaling=2^0
  Out1 : Outport  OutDataType=fixdt(1, 16)  OutScaling=2^0
  Out2 : Outport  Port=2  OutDataType=fixdt(1, 16)  OutScaling=2^0
  wires:
  In/1 -> Out1/1, Out2/1

== system receiver_overall_reset/Receiver/Sym-Chooser/6-14/Corr0/Delay_Line/DE10/1to2 ==
  In : Inport  OutDataType=fixdt(1, 16)  OutScaling=2^0
  Out1 : Outport  OutDataType=fixdt(1, 16)  OutScaling=2^0
  Out2 : Outport  Port=2  OutDataType=fixdt(1, 16)  OutScaling=2^0
  wires:
  In/1 -> Out2/1, Out1/1

== system receiver_overall_reset/Receiver/Sym-Chooser/6-14/Corr0/Delay_Line/DE11/1to2 ==
  In : Inport  OutDataType=fixdt(1, 16)  OutScaling=2^0
  Out1 : Outport  OutDataType=fixdt(1, 16)  OutScaling=2^0
  Out2 : Outport  Port=2  OutDataType=fixdt(1, 16)  OutScaling=2^0
  wires:
  In/1 -> Out2/1, Out1/1

== system receiver_overall_reset/Receiver/Sym-Chooser/6-14/Corr0/Delay_Line/DE12/1to2 ==
  In : Inport  OutDataType=fixdt(1, 16)  OutScaling=2^0
  Out1 : Outport  OutDataType=fixdt(1, 16)  OutScaling=2^0
  Out2 : Outport  Port=2  OutDataType=fixdt(1, 16)  OutScaling=2^0
  wires:
  In/1 -> Out2/1, Out1/1

== system receiver_overall_reset/Receiver/Sym-Chooser/6-14/Corr0/Delay_Line/DE13/1to2 ==
  In : Inport  OutDataType=fixdt(1, 16)  OutScaling=2^0
  Out1 : Outport  OutDataType=fixdt(1, 16)  OutScaling=2^0
  Out2 : Outport  Port=2  OutDataType=fixdt(1, 16)  OutScaling=2^0
  wires:
  In/1 -> Out2/1, Out1/1

== system receiver_overall_reset/Receiver/Sym-Chooser/6-14/Corr0/Delay_Line/DE14/1to2 ==
  In : Inport  OutDataType=fixdt(1, 16)  OutScaling=2^0
  Out1 : Outport  OutDataType=fixdt(1, 16)  OutScaling=2^0
  Out2 : Outport  Port=2  OutDataType=fixdt(1, 16)  OutScaling=2^0
  wires:
  In/1 -> Out2/1, Out1/1

== system receiver_overall_reset/Receiver/Sym-Chooser/6-14/Corr0/Delay_Line/DE15/1to2 ==
  In : Inport  OutDataType=fixdt(1, 16)  OutScaling=2^0
  Out1 : Outport  OutDataType=fixdt(1, 16)  OutScaling=2^0
  Out2 : Outport  Port=2  OutDataType=fixdt(1, 16)  OutScaling=2^0
  wires:
  In/1 -> Out2/1, Out1/1

== system receiver_overall_reset/Receiver/Sym-Chooser/6-14/Corr0/Delay_Line/DE16/1to2 ==
  In : Inport  OutDataType=fixdt(1, 16)  OutScaling=2^0
  Out1 : Outport  OutDataType=fixdt(1, 16)  OutScaling=2^0
  Out2 : Outport  Port=2  OutDataType=fixdt(1, 16)  OutScaling=2^0
  wires:
  In/1 -> Out2/1, Out1/1

== system receiver_overall_reset/Receiver/Sym-Chooser/6-14/Corr0/Delay_Line/DE17/1to2 ==
  In : Inport  OutDataType=fixdt(1, 16)  OutScaling=2^0
  Out1 : Outport  OutDataType=fixdt(1, 16)  OutScaling=2^0
  Out2 : Outport  Port=2  OutDataType=fixdt(1, 16)  OutScaling=2^0
  wires:
  In/1 -> Out2/1, Out1/1

== system receiver_overall_reset/Receiver/Sym-Chooser/6-14/Corr0/Delay_Line/DE18/1to2 ==
  In : Inport  OutDataType=fixdt(1, 16)  OutScaling=2^0
  Out1 : Outport  OutDataType=fixdt(1, 16)  OutScaling=2^0
  Out2 : Outport  Port=2  OutDataType=fixdt(1, 16)  OutScaling=2^0
  wires:
  In/1 -> Out2/1, Out1/1

== system receiver_overall_reset/Receiver/Sym-Chooser/6-14/Corr0/Delay_Line/DE19/1to2 ==
  In : Inport  OutDataType=fixdt(1, 16)  OutScaling=2^0
  Out1 : Outport  OutDataType=fixdt(1, 16)  OutScaling=2^0
  Out2 : Outport  Port=2  OutDataType=fixdt(1, 16)  OutScaling=2^0
  wires:
  In/1 -> Out2/1, Out1/1

== system receiver_overall_reset/Receiver/Sym-Chooser/6-14/Corr0/Delay_Line/DE2/1to2 ==
  In : Inport  OutDataType=fixdt(1, 16)  OutScaling=2^0
  Out1 : Outport  OutDataType=fixdt(1, 16)  OutScaling=2^0
  Out2 : Outport  Port=2  OutDataType=fixdt(1, 16)  OutScaling=2^0
  wires:
  In/1 -> Out2/1, Out1/1

== system receiver_overall_reset/Receiver/Sym-Chooser/6-14/Corr0/Delay_Line/DE20/1to2 ==
  In : Inport  OutDataType=fixdt(1, 16)  OutScaling=2^0
  Out1 : Outport  OutDataType=fixdt(1, 16)  OutScaling=2^0
  Out2 : Outport  Port=2  OutDataType=fixdt(1, 16)  OutScaling=2^0
  wires:
  In/1 -> Out2/1, Out1/1

== system receiver_overall_reset/Receiver/Sym-Chooser/6-14/Corr0/Delay_Line/DE21/1to2 ==
  In : Inport  OutDataType=fixdt(1, 16)  OutScaling=2^0
  Out1 : Outport  OutDataType=fixdt(1, 16)  OutScaling=2^0
  Out2 : Outport  Port=2  OutDataType=fixdt(1, 16)  OutScaling=2^0
  wires:
  In/1 -> Out2/1, Out1/1

== system receiver_overall_reset/Receiver/Sym-Chooser/6-14/Corr0/Delay_Line/DE22/1to2 ==
  In : Inport  OutDataType=fixdt(1, 16)  OutScaling=2^0
  Out1 : Outport  OutDataType=fixdt(1, 16)  OutScaling=2^0
  Out2 : Outport  Port=2  OutDataType=fixdt(1, 16)  OutScaling=2^0
  wires:
  In/1 -> Out2/1, Out1/1

== system receiver_overall_reset/Receiver/Sym-Chooser/6-14/Corr0/Delay_Line/DE23/1to2 ==
  In : Inport  OutDataType=fixdt(1, 16)  OutScaling=2^0
  Out1 : Outport  OutDataType=fixdt(1, 16)  OutScaling=2^0
  Out2 : Outport  Port=2  OutDataType=fixdt(1, 16)  OutScaling=2^0
  wires:
  In/1 -> Out2/1, Out1/1

== system receiver_overall_reset/Receiver/Sym-Chooser/6-14/Corr0/Delay_Line/DE24/1to2 ==
  In : Inport  OutDataType=fixdt(1, 16)  OutScaling=2^0
  Out1 : Outport  OutDataType=fixdt(1, 16)  OutScaling=2^0
  Out2 : Outport  Port=2  OutDataType=fixdt(1, 16)  OutScaling=2^0
  wires:
  In/1 -> Out2/1, Out1/1

== system receiver_overall_reset/Receiver/Sym-Chooser/6-14/Corr0/Delay_Line/DE25/1to2 ==
  In : Inport  OutDataType=fixdt(1, 16)  OutScaling=2^0
  Out1 : Outport  OutDataType=fixdt(1, 16)  OutScaling=2^0
  Out2 : Outport  Port=2  OutDataType=fixdt(1, 16)  OutScaling=2^0
  wires:
  In/1 -> Out2/1, Out1/1

== system receiver_overall_reset/Receiver/Sym-Chooser/6-14/Corr0/Delay_Line/DE26/1to2 ==
  In : Inport  OutDataType=fixdt(1, 16)  OutScaling=2^0
  Out1 : Outport  OutDataType=fixdt(1, 16)  OutScaling=2^0
  Out2 : Outport  Port=2  OutDataType=fixdt(1, 16)  OutScaling=2^0
  wires:
  In/1 -> Out2/1, Out1/1

== system receiver_overall_reset/Receiver/Sym-Chooser/6-14/Corr0/Delay_Line/DE27/1to2 ==
  In : Inport  OutDataType=fixdt(1, 16)  OutScaling=2^0
  Out1 : Outport  OutDataType=fixdt(1, 16)  OutScaling=2^0
  Out2 : Outport  Port=2  OutDataType=fixdt(1, 16)  OutScaling=2^0
  wires:
  In/1 -> Out2/1, Out1/1

== system receiver_overall_reset/Receiver/Sym-Chooser/6-14/Corr0/Delay_Line/DE28/1to2 ==
  In : Inport  OutDataType=fixdt(1, 16)  OutScaling=2^0
  Out1 : Outport  OutDataType=fixdt(1, 16)  OutScaling=2^0
  Out2 : Outport  Port=2  OutDataType=fixdt(1, 16)  OutScaling=2^0
  wires:
  In/1 -> Out2/1, Out1/1

== system receiver_overall_reset/Receiver/Sym-Chooser/6-14/Corr0/Delay_Line/DE29/1to2 ==
  In : Inport  OutDataType=fixdt(1, 16)  OutScaling=2^0
  Out1 : Outport  OutDataType=fixdt(1, 16)  OutScaling=2^0
  Out2 : Outport  Port=2  OutDataType=fixdt(1, 16)  OutScaling=2^0
  wires:
  In/1 -> Out2/1, Out1/1

== system receiver_overall_reset/Receiver/Sym-Chooser/6-14/Corr0/Delay_Line/DE3/1to2 ==
  In : Inport  OutDataType=fixdt(1, 16)  OutScaling=2^0
  Out1 : Outport  OutDataType=fixdt(1, 16)  OutScaling=2^0
  Out2 : Outport  Port=2  OutDataType=fixdt(1, 16)  OutScaling=2^0
  wires:
  In/1 -> Out2/1, Out1/1

== system receiver_overall_reset/Receiver/Sym-Chooser/6-14/Corr0/Delay_Line/DE30/1to2 ==
  In : Inport  OutDataType=fixdt(1, 16)  OutScaling=2^0
  Out1 : Outport  OutDataType=fixdt(1, 16)  OutScaling=2^0
  Out2 : Outport  Port=2  OutDataType=fixdt(1, 16)  OutScaling=2^0
  wires:
  In/1 -> Out2/1, Out1/1

== system receiver_overall_reset/Receiver/Sym-Chooser/6-14/Corr0/Delay_Line/DE4/1to2 ==
  In : Inport  OutDataType=fixdt(1, 16)  OutScaling=2^0
  Out1 : Outport  OutDataType=fixdt(1, 16)  OutScaling=2^0
  Out2 : Outport  Port=2  OutDataType=fixdt(1, 16)  OutScaling=2^0
  wires:
  In/1 -> Out2/1, Out1/1

== system receiver_overall_reset/Receiver/Sym-Chooser/6-14/Corr0/Delay_Line/DE5/1to2 ==
  In : Inport  OutDataType=fixdt(1, 16)  OutScaling=2^0
  Out1 : Outport  OutDataType=fixdt(1, 16)  OutScaling=2^0
  Out2 : Outport  Port=2  OutDataType=fixdt(1, 16)  OutScaling=2^0
  wires:
  In/1 -> Out2/1, Out1/1

== system receiver_overall_reset/Receiver/Sym-Chooser/6-14/Corr0/Delay_Line/DE6/1to2 ==
  In : Inport  OutDataType=fixdt(1, 16)  OutScaling=2^0
  Out1 : Outport  OutDataType=fixdt(1, 16)  OutScaling=2^0
  Out2 : Outport  Port=2  OutDataType=fixdt(1, 16)  OutScaling=2^0
  wires:
  In/1 -> Out2/1, Out1/1

== system receiver_overall_reset/Receiver/Sym-Chooser/6-14/Corr0/Delay_Line/DE7/1to2 ==
  In : Inport  OutDataType=fixdt(1, 16)  OutScaling=2^0
  Out1 : Outport  OutDataType=fixdt(1, 16)  OutScaling=2^0
  Out2 : Outport  Port=2  OutDataType=fixdt(1, 16)  OutScaling=2^0
  wires:
  In/1 -> Out2/1, Out1/1

== system receiver_overall_reset/Receiver/Sym-Chooser/6-14/Corr0/Delay_Line/DE8/1to2 ==
  In : Inport  OutDataType=fixdt(1, 16)  OutScaling=2^0
  Out1 : Outport  OutDataType=fixdt(1, 16)  OutScaling=2^0
  Out2 : Outport  Port=2  OutDataType=fixdt(1, 16)  OutScaling=2^0
  wires:
  In/1 -> Out2/1, Out1/1

== system receiver_overall_reset/Receiver/Sym-Chooser/6-14/Corr0/Delay_Line/DE9/1to2 ==
  In : Inport  OutDataType=fixdt(1, 16)  OutScaling=2^0
  Out1 : Outport  OutDataType=fixdt(1, 16)  OutScaling=2^0
  Out2 : Outport  Port=2  OutDataType=fixdt(1, 16)  OutScaling=2^0
  wires:
  In/1 -> Out2/1, Out1/1

== system receiver_overall_reset/Receiver/Sym-Chooser/7-15/Corr0/Delay_Line/DE1/1to2 ==
  In : Inport  OutDataType=fixdt(1, 16)  OutScaling=2^0
  Out1 : Outport  OutDataType=fixdt(1, 16)  OutScaling=2^0
  Out2 : Outport  Port=2  OutDataType=fixdt(1, 16)  OutScaling=2^0
  wires:
  In/1 -> Out1/1, Out2/1

== system receiver_overall_reset/Receiver/Sym-Chooser/7-15/Corr0/Delay_Line/DE10/1to2 ==
  In : Inport  OutDataType=fixdt(1, 16)  OutScaling=2^0
  Out1 : Outport  OutDataType=fixdt(1, 16)  OutScaling=2^0
  Out2 : Outport  Port=2  OutDataType=fixdt(1, 16)  OutScaling=2^0
  wires:
  In/1 -> Out2/1, Out1/1

== system receiver_overall_reset/Receiver/Sym-Chooser/7-15/Corr0/Delay_Line/DE11/1to2 ==
  In : Inport  OutDataType=fixdt(1, 16)  OutScaling=2^0
  Out1 : Outport  OutDataType=fixdt(1, 16)  OutScaling=2^0
  Out2 : Outport  Port=2  OutDataType=fixdt(1, 16)  OutScaling=2^0
  wires:
  In/1 -> Out2/1, Out1/1

== system receiver_overall_reset/Receiver/Sym-Chooser/7-15/Corr0/Delay_Line/DE12/1to2 ==
  In : Inport  OutDataType=fixdt(1, 16)  OutScaling=2^0
  Out1 : Outport  OutDataType=fixdt(1, 16)  OutScaling=2^0
  Out2 : Outport  Port=2  OutDataType=fixdt(1, 16)  OutScaling=2^0
  wires:
  In/1 -> Out2/1, Out1/1

== system receiver_overall_reset/Receiver/Sym-Chooser/7-15/Corr0/Delay_Line/DE13/1to2 ==
  In : Inport  OutDataType=fixdt(1, 16)  OutScaling=2^0
  Out1 : Outport  OutDataType=fixdt(1, 16)  OutScaling=2^0
  Out2 : Outport  Port=2  OutDataType=fixdt(1, 16)  OutScaling=2^0
  wires:
  In/1 -> Out2/1, Out1/1

== system receiver_overall_reset/Receiver/Sym-Chooser/7-15/Corr0/Delay_Line/DE14/1to2 ==
  In : Inport  OutDataType=fixdt(1, 16)  OutScaling=2^0
  Out1 : Outport  OutDataType=fixdt(1, 16)  OutScaling=2^0
  Out2 : Outport  Port=2  OutDataType=fixdt(1, 16)  OutScaling=2^0
  wires:
  In/1 -> Out2/1, Out1/1

== system receiver_overall_reset/Receiver/Sym-Chooser/7-15/Corr0/Delay_Line/DE15/1to2 ==
  In : Inport  OutDataType=fixdt(1, 16)  OutScaling=2^0
  Out1 : Outport  OutDataType=fixdt(1, 16)  OutScaling=2^0
  Out2 : Outport  Port=2  OutDataType=fixdt(1, 16)  OutScaling=2^0
  wires:
  In/1 -> Out2/1, Out1/1

== system receiver_overall_reset/Receiver/Sym-Chooser/7-15/Corr0/Delay_Line/DE16/1to2 ==
  In : Inport  OutDataType=fixdt(1, 16)  OutScaling=2^0
  Out1 : Outport  OutDataType=fixdt(1, 16)  OutScaling=2^0
  Out2 : Outport  Port=2  OutDataType=fixdt(1, 16)  OutScaling=2^0
  wires:
  In/1 -> Out2/1, Out1/1

== system receiver_overall_reset/Receiver/Sym-Chooser/7-15/Corr0/Delay_Line/DE17/1to2 ==
  In : Inport  OutDataType=fixdt(1, 16)  OutScaling=2^0
  Out1 : Outport  OutDataType=fixdt(1, 16)  OutScaling=2^0
  Out2 : Outport  Port=2  OutDataType=fixdt(1, 16)  OutScaling=2^0
  wires:
  In/1 -> Out2/1, Out1/1

== system receiver_overall_reset/Receiver/Sym-Chooser/7-15/Corr0/Delay_Line/DE18/1to2 ==
  In : Inport  OutDataType=fixdt(1, 16)  OutScaling=2^0
  Out1 : Outport  OutDataType=fixdt(1, 16)  OutScaling=2^0
  Out2 : Outport  Port=2  OutDataType=fixdt(1, 16)  OutScaling=2^0
  wires:
  In/1 -> Out2/1, Out1/1

== system receiver_overall_reset/Receiver/Sym-Chooser/7-15/Corr0/Delay_Line/DE19/1to2 ==
  In : Inport  OutDataType=fixdt(1, 16)  OutScaling=2^0
  Out1 : Outport  OutDataType=fixdt(1, 16)  OutScaling=2^0
  Out2 : Outport  Port=2  OutDataType=fixdt(1, 16)  OutScaling=2^0
  wires:
  In/1 -> Out2/1, Out1/1

== system receiver_overall_reset/Receiver/Sym-Chooser/7-15/Corr0/Delay_Line/DE2/1to2 ==
  In : Inport  OutDataType=fixdt(1, 16)  OutScaling=2^0
  Out1 : Outport  OutDataType=fixdt(1, 16)  OutScaling=2^0
  Out2 : Outport  Port=2  OutDataType=fixdt(1, 16)  OutScaling=2^0
  wires:
  In/1 -> Out2/1, Out1/1

== system receiver_overall_reset/Receiver/Sym-Chooser/7-15/Corr0/Delay_Line/DE20/1to2 ==
  In : Inport  OutDataType=fixdt(1, 16)  OutScaling=2^0
  Out1 : Outport  OutDataType=fixdt(1, 16)  OutScaling=2^0
  Out2 : Outport  Port=2  OutDataType=fixdt(1, 16)  OutScaling=2^0
  wires:
  In/1 -> Out2/1, Out1/1

== system receiver_overall_reset/Receiver/Sym-Chooser/7-15/Corr0/Delay_Line/DE21/1to2 ==
  In : Inport  OutDataType=fixdt(1, 16)  OutScaling=2^0
  Out1 : Outport  OutDataType=fixdt(1, 16)  OutScaling=2^0
  Out2 : Outport  Port=2  OutDataType=fixdt(1, 16)  OutScaling=2^0
  wires:
  In/1 -> Out2/1, Out1/1

== system receiver_overall_reset/Receiver/Sym-Chooser/7-15/Corr0/Delay_Line/DE22/1to2 ==
  In : Inport  OutDataType=fixdt(1, 16)  OutScaling=2^0
  Out1 : Outport  OutDataType=fixdt(1, 16)  OutScaling=2^0
  Out2 : Outport  Port=2  OutDataType=fixdt(1, 16)  OutScaling=2^0
  wires:
  In/1 -> Out2/1, Out1/1

== system receiver_overall_reset/Receiver/Sym-Chooser/7-15/Corr0/Delay_Line/DE23/1to2 ==
  In : Inport  OutDataType=fixdt(1, 16)  OutScaling=2^0
  Out1 : Outport  OutDataType=fixdt(1, 16)  OutScaling=2^0
  Out2 : Outport  Port=2  OutDataType=fixdt(1, 16)  OutScaling=2^0
  wires:
  In/1 -> Out2/1, Out1/1

== system receiver_overall_reset/Receiver/Sym-Chooser/7-15/Corr0/Delay_Line/DE24/1to2 ==
  In : Inport  OutDataType=fixdt(1, 16)  OutScaling=2^0
  Out1 : Outport  OutDataType=fixdt(1, 16)  OutScaling=2^0
  Out2 : Outport  Port=2  OutDataType=fixdt(1, 16)  OutScaling=2^0
  wires:
  In/1 -> Out2/1, Out1/1

== system receiver_overall_reset/Receiver/Sym-Chooser/7-15/Corr0/Delay_Line/DE25/1to2 ==
  In : Inport  OutDataType=fixdt(1, 16)  OutScaling=2^0
  Out1 : Outport  OutDataType=fixdt(1, 16)  OutScaling=2^0
  Out2 : Outport  Port=2  OutDataType=fixdt(1, 16)  OutScaling=2^0
  wires:
  In/1 -> Out2/1, Out1/1

== system receiver_overall_reset/Receiver/Sym-Chooser/7-15/Corr0/Delay_Line/DE26/1to2 ==
  In : Inport  OutDataType=fixdt(1, 16)  OutScaling=2^0
  Out1 : Outport  OutDataType=fixdt(1, 16)  OutScaling=2^0
  Out2 : Outport  Port=2  OutDataType=fixdt(1, 16)  OutScaling=2^0
  wires:
  In/1 -> Out2/1, Out1/1

== system receiver_overall_reset/Receiver/Sym-Chooser/7-15/Corr0/Delay_Line/DE27/1to2 ==
  In : Inport  OutDataType=fixdt(1, 16)  OutScaling=2^0
  Out1 : Outport  OutDataType=fixdt(1, 16)  OutScaling=2^0
  Out2 : Outport  Port=2  OutDataType=fixdt(1, 16)  OutScaling=2^0
  wires:
  In/1 -> Out2/1, Out1/1

== system receiver_overall_reset/Receiver/Sym-Chooser/7-15/Corr0/Delay_Line/DE28/1to2 ==
  In : Inport  OutDataType=fixdt(1, 16)  OutScaling=2^0
  Out1 : Outport  OutDataType=fixdt(1, 16)  OutScaling=2^0
  Out2 : Outport  Port=2  OutDataType=fixdt(1, 16)  OutScaling=2^0
  wires:
  In/1 -> Out2/1, Out1/1

== system receiver_overall_reset/Receiver/Sym-Chooser/7-15/Corr0/Delay_Line/DE29/1to2 ==
  In : Inport  OutDataType=fixdt(1, 16)  OutScaling=2^0
  Out1 : Outport  OutDataType=fixdt(1, 16)  OutScaling=2^0
  Out2 : Outport  Port=2  OutDataType=fixdt(1, 16)  OutScaling=2^0
  wires:
  In/1 -> Out2/1, Out1/1

== system receiver_overall_reset/Receiver/Sym-Chooser/7-15/Corr0/Delay_Line/DE3/1to2 ==
  In : Inport  OutDataType=fixdt(1, 16)  OutScaling=2^0
  Out1 : Outport  OutDataType=fixdt(1, 16)  OutScaling=2^0
  Out2 : Outport  Port=2  OutDataType=fixdt(1, 16)  OutScaling=2^0
  wires:
  In/1 -> Out2/1, Out1/1

== system receiver_overall_reset/Receiver/Sym-Chooser/7-15/Corr0/Delay_Line/DE30/1to2 ==
  In : Inport  OutDataType=fixdt(1, 16)  OutScaling=2^0
  Out1 : Outport  OutDataType=fixdt(1, 16)  OutScaling=2^0
  Out2 : Outport  Port=2  OutDataType=fixdt(1, 16)  OutScaling=2^0
  wires:
  In/1 -> Out2/1, Out1/1

== system receiver_overall_reset/Receiver/Sym-Chooser/7-15/Corr0/Delay_Line/DE4/1to2 ==
  In : Inport  OutDataType=fixdt(1, 16)  OutScaling=2^0
  Out1 : Outport  OutDataType=fixdt(1, 16)  OutScaling=2^0
  Out2 : Outport  Port=2  OutDataType=fixdt(1, 16)  OutScaling=2^0
  wires:
  In/1 -> Out2/1, Out1/1

== system receiver_overall_reset/Receiver/Sym-Chooser/7-15/Corr0/Delay_Line/DE5/1to2 ==
  In : Inport  OutDataType=fixdt(1, 16)  OutScaling=2^0
  Out1 : Outport  OutDataType=fixdt(1, 16)  OutScaling=2^0
  Out2 : Outport  Port=2  OutDataType=fixdt(1, 16)  OutScaling=2^0
  wires:
  In/1 -> Out2/1, Out1/1

== system receiver_overall_reset/Receiver/Sym-Chooser/7-15/Corr0/Delay_Line/DE6/1to2 ==
  In : Inport  OutDataType=fixdt(1, 16)  OutScaling=2^0
  Out1 : Outport  OutDataType=fixdt(1, 16)  OutScaling=2^0
  Out2 : Outport  Port=2  OutDataType=fixdt(1, 16)  OutScaling=2^0
  wires:
  In/1 -> Out2/1, Out1/1

== system receiver_overall_reset/Receiver/Sym-Chooser/7-15/Corr0/Delay_Line/DE7/1to2 ==
  In : Inport  OutDataType=fixdt(1, 16)  OutScaling=2^0
  Out1 : Outport  OutDataType=fixdt(1, 16)  OutScaling=2^0
  Out2 : Outport  Port=2  OutDataType=fixdt(1, 16)  OutScaling=2^0
  wires:
  In/1 -> Out2/1, Out1/1

== system receiver_overall_reset/Receiver/Sym-Chooser/7-15/Corr0/Delay_Line/DE8/1to2 ==
  In : Inport  OutDataType=fixdt(1, 16)  OutScaling=2^0
  Out1 : Outport  OutDataType=fixdt(1, 16)  OutScaling=2^0
  Out2 : Outport  Port=2  OutDataType=fixdt(1, 16)  OutScaling=2^0
  wires:
  In/1 -> Out2/1, Out1/1

== system receiver_overall_reset/Receiver/Sym-Chooser/7-15/Corr0/Delay_Line/DE9/1to2 ==
  In : Inport  OutDataType=fixdt(1, 16)  OutScaling=2^0
  Out1 : Outport  OutDataType=fixdt(1, 16)  OutScaling=2^0
  Out2 : Outport  Port=2  OutDataType=fixdt(1, 16)  OutScaling=2^0
  wires:
  In/1 -> Out2/1, Out1/1
